simulink model "linio_nochmal_nur_CC"  (R2013a)
settings: Solver=ode45  StartTime=0.0  StopTime=10.0  MaxStep=1e-4  RelTol=1e-3
undefined symbols (not defined in the file or in its folder): Lc, Rc, Rsh
libraries: simulink x1
settings Model: Creator=mainster  LastModifiedBy=mainster

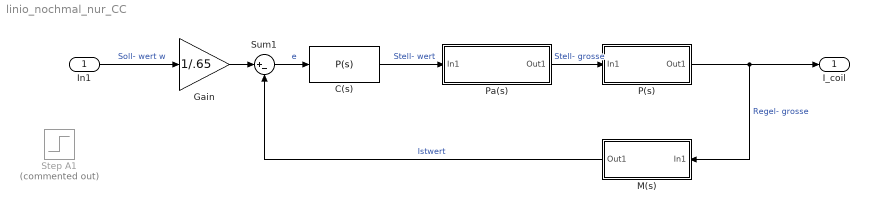
== system linio_nochmal_nur_CC ==
  In1 : Inport
  C(s) : simulink/Continuous/PID Controller  Controller=P  TimeDomain=Continuous-time  SampleTime=-1  IntegratorMethod=Forward Euler  FilterMethod=Forward Euler  Form=Ideal  P=20  I=14078.2261040339  D=0  N=100  InitialConditionSource=internal  InitialConditionForIntegrator=0  InitialConditionForFilter=0  ExternalReset=none  LimitOutput=off  UpperSaturationLimit=inf  LowerSaturationLimit=-inf  LinearizeAsGain=on  AntiWindupMode=none  Kb=1  TrackingMode=off  Kt=1  PParamMin=[]  PParamMax=[]  IParamMin=[]  IParamMax=[]  DParamMin=[]  DParamMax=[]  NParamMin=[]  NParamMax=[]  KbParamMin=[]  KbParamMax=[]  KtParamMin=[]  KtParamMax=[]  POutMin=[]  POutMax=[]  IOutMin=[]  IOutMax=[]  DOutMin=[]  DOutMax=[]  NOutMin=[]  NOutMax=[]  KbOutMin=[]  KbOutMax=[]  KtOutMin=[]  KtOutMax=[]  IntegratorOutMin=[]  IntegratorOutMax=[]  FilterOutMin=[]  FilterOutMax=[]  SumOutMin=[]  SumOutMax=[]  SumI1OutMin=[]  SumI1OutMax=[]  SumI2OutMin=[]  SumI2OutMax=[]  SumI3OutMin=[]  SumI3OutMax=[]  SumDOutMin=[]  SumDOutMax=[]  SaturationOutMin=[]  SaturationOutMax=[]  IntegratorContinuousStateAttributes=''  IntegratorStateMustResolveToSignalObject=off  IntegratorRTWStateStorageClass=Auto  FilterContinuousStateAttributes=''  FilterStateMustResolveToSignalObject=off  FilterRTWStateStorageClass=Auto  mask(PID 1dof){}
      mask Display:
      | % This is a new mask on top of the base mask.
      | % Use "View base mask" link below to see the base mask.
      | 
      | disp('Regler')
  Gain : Gain  Gain=1/.65
  M(s) : Subsystem
      mask Display: disp('Messwandler\nSensor')
  P(s) : Subsystem
      mask Display: disp('Regelstrecke\nPlant')
  Pa(s) : Subsystem
      mask Display: disp('Stellglied\nPlant actuator')
  Step A1 : Step  Commented=on  Time=1e-3  After=0  SampleTime=0  ZeroCross=off
      settings: AttributesFormatString=Ampl.: %<After>\ntime:%<Time>
  Sum1 : Sum  Inputs=|+-
  I_coil : Outport
  wires:
  Sum1/1 -> C(s)/1  "e"
  C(s)/1 -> Pa(s)/1(In1)  "Stell- wert"
  Pa(s)/1(Out1) -> P(s)/1(In1)  "Stell- grosse"
  P(s)/1(Out1) -> M(s)/1(In1), I_coil/1  "Regel- grosse"
  M(s)/1(Out1) -> Sum1/2  "Istwert"
  Gain/1 -> Sum1/1
  In1/1 -> Gain/1  "Soll- wert w"

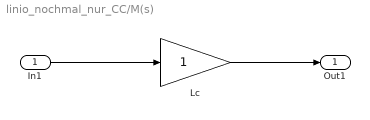
== system linio_nochmal_nur_CC/M(s) ==
  In1 : Inport
  Lc : Gain
  Out1 : Outport
  wires:
  In1/1 -> Lc/1
  Lc/1 -> Out1/1

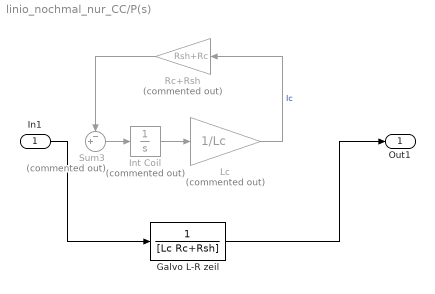
== system linio_nochmal_nur_CC/P(s) ==
  In1 : Inport
  Galvo L-R zeil : TransferFcn  Numerator=1  Denominator=[Lc Rc+Rsh]
  Int Coil : Integrator  Commented=on
  Lc : Gain  Commented=on  Gain=1/Lc
  Rc+Rsh : Gain  Commented=on  Gain=Rsh+Rc
  Sum3 : Sum  Commented=on  Inputs=-+|
  Out1 : Outport
  wires:
  In1/1 -> Galvo L-R zeil/1
  Sum3/1 -> Int Coil/1
  Int Coil/1 -> Lc/1
  Lc/1 -> Rc+Rsh/1  "Ic"
  Rc+Rsh/1 -> Sum3/1
  Galvo L-R zeil/1 -> Out1/1

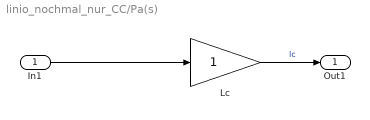
== system linio_nochmal_nur_CC/Pa(s) ==
  In1 : Inport
  Lc : Gain
  Out1 : Outport
  wires:
  In1/1 -> Lc/1
  Lc/1 -> Out1/1  "Ic"
